simulink model "backstepping_handle_statico_last"  (R2018b)
settings: Solver=VariableStepAuto  StartTime=0.0  StopTime=10  RelTol=1e-3
values from neighbouring files (symbols this model uses):
  cond_init = [0, 150/180*pi, pi/3, -pi/2, -3*pi/4,-150/180*pi]'    [init.m]
  hand_des = p(6,:)'    [init.m]
  Law_param = [kd,kd,kd,kd,kd,kd ... (first row only)    [LAUNCH_Backstepping.m]    (also in LAUNCH_Backstepping_Adaptavive.m = [kp,kp,kp,kp,kp,kp; LAUNCH_PD_TRAJ.m = [300000,300000,300000,300000,300000,300000)
  param = param'    [init.m]
settings Model: Creator=Utente  LastModifiedBy=Utente

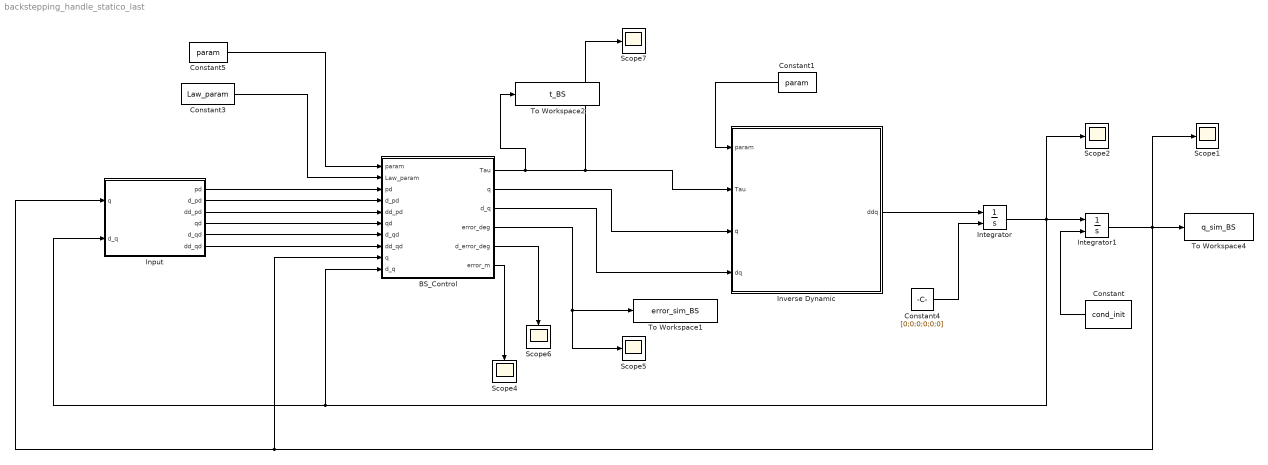
== system backstepping_handle_statico_last ==
  BS_Control : MATLAB Function  TreatAsAtomicUnit=on
  Constant : Constant  Value=cond_init
  Constant1 : Constant  Value=param
  Constant3 : Constant  Value=Law_param
  Constant4 : Constant  Value=[0;0;0;0;0;0]
  Constant5 : Constant  Value=param
  Input : Subsystem
  Integrator : Integrator  InitialConditionSource=external  InitialCondition=[0;0;0;0;0;0]
  Integrator1 : Integrator  InitialConditionSource=external
  Inverse Dynamic : MATLAB Function  TreatAsAtomicUnit=on
  Scope{1..2,4..7} (6 alike) : Scope
  To Workspace1 : ToWorkspace  VariableName=error_sim_BS  SaveFormat=Structure With Time  SampleTime=-1
      settings: Save2DSignal=2-D array (concatenate along first dimension)
  To Workspace2 : ToWorkspace  VariableName=t_BS  SaveFormat=Structure With Time  SampleTime=-1
      settings: Save2DSignal=2-D array (concatenate along first dimension)
  To Workspace4 : ToWorkspace  VariableName=q_sim_BS  SaveFormat=Structure With Time  SampleTime=-1
      settings: Save2DSignal=2-D array (concatenate along first dimension)
  wires:
  Constant5/1 -> BS_Control/1(param)
  Constant3/1 -> BS_Control/2(Law_param)
  BS_Control/2(q) -> Inverse Dynamic/3(q)
  BS_Control/3(d_q) -> Inverse Dynamic/4(dq)
  Constant4/1 -> Integrator/2
  Integrator/1 -> BS_Control/10("d_q "), Input/2(d_q), Integrator1/1, Scope2/1
  Integrator1/1 -> Input/1(q), BS_Control/9("q "), To Workspace4/1, Scope1/1
  Inverse Dynamic/1(ddq) -> Integrator/1
  Constant/1 -> Integrator1/2
  Constant1/1 -> Inverse Dynamic/1(param)
  BS_Control/4(error_deg) -> Scope5/1, To Workspace1/1
  BS_Control/5(d_error_deg) -> Scope6/1
  Input/4(qd) -> BS_Control/6(qd)
  Input/5(d_qd) -> BS_Control/7(d_qd)
  Input/6(dd_qd) -> BS_Control/8(dd_qd)
  Input/3(dd_pd) -> BS_Control/5(dd_pd)
  Input/2(d_pd) -> BS_Control/4(d_pd)
  Input/1(pd) -> BS_Control/3(pd)
  BS_Control/6(error_m) -> Scope4/1
  BS_Control/1(Tau) -> To Workspace2/1, Scope7/1, Inverse Dynamic/2(Tau)

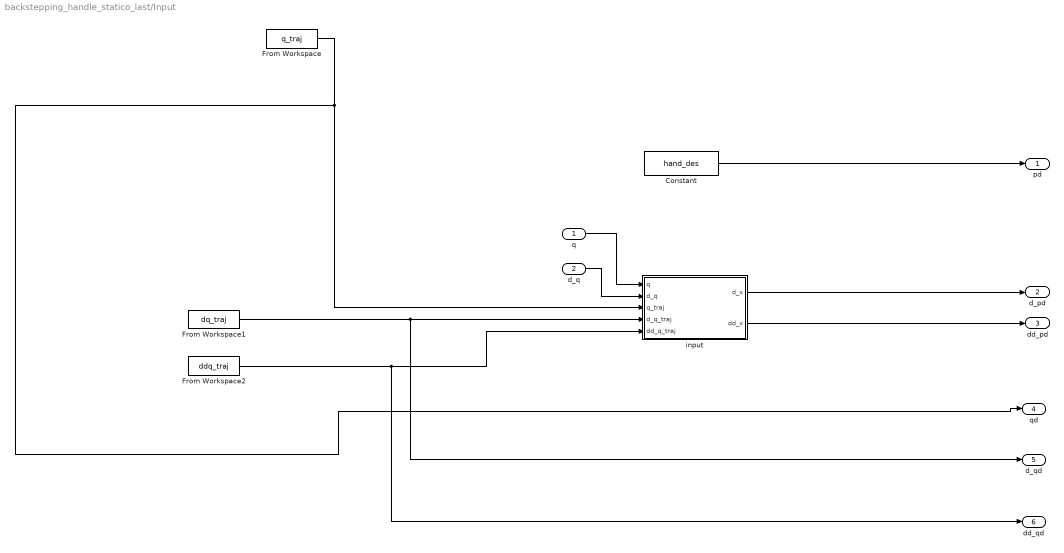
== system backstepping_handle_statico_last/Input ==
  q : Inport
  d_q : Inport  Port=2
  Constant : Constant  Value=hand_des
  From Workspace : FromWorkspace  VariableName=q_traj  SampleTime=0
  From Workspace1 : FromWorkspace  VariableName=dq_traj  SampleTime=0
  From Workspace2 : FromWorkspace  VariableName=ddq_traj  SampleTime=0
  "input " : MATLAB Function  TreatAsAtomicUnit=on
  pd : Outport
  d_pd : Outport  Port=2
  dd_pd : Outport  Port=3
  qd : Outport  Port=4
  d_qd : Outport  Port=5
  dd_qd : Outport  Port=6
  wires:
  From Workspace/1 -> "input "/3(q_traj), qd/1
  From Workspace1/1 -> d_qd/1, "input "/4(d_q_traj)
  From Workspace2/1 -> dd_qd/1, "input "/5(dd_q_traj)
  q/1 -> "input "/1(q)
  d_q/1 -> "input "/2(d_q)
  "input "/1(d_x) -> d_pd/1
  "input "/2(dd_x) -> dd_pd/1
  Constant/1 -> pd/1

== matlab function backstepping_handle_statico_last/BS_Control ==
  data: param input; Tau output; Law_param input; pd input; d_pd input; dd_pd input; qd input; d_qd input; dd_qd input; q input; d_q input; q output; d_q output; error_deg output; d_error_deg output; error_m output
function [Tau, q, d_q, error_deg, d_error_deg, error_m] = BS_Control(param, Law_param, pd, d_pd, dd_pd,qd, d_qd, dd_qd, q, d_q)


    [B,C,G] = Dinamica_new(param,q,d_q);
    
    JHand = J_hand_fun(q);
    pinv_JHand = pinv(JHand);
    
    [p,~,~] = Direct_Kinematics(param,q);
    
    d_Jhand = d_Jhand_fun(q,d_q);
    pinv_d_JHand = pinv(d_Jhand);
    
    Kd = Law_param(1,1)*eye(6);
    L = Law_param(2,1)*eye(6);
    e = qd - q;
    d_e = d_qd - d_q;
    
    d_qr = d_qd + L*e;
    dd_qr = dd_qd + L*d_e;

    s = d_qr - d_q;   
    
    Tau = B*dd_qr + C*d_qr + G + Kd*s + e;

    %SPAZIO TASK
%     Kd = Law_param(1,1)*eye(6);
%     L = Law_param(2,1)*eye(3);
% 
%     e = pd - p(6,:)';
%     d_e = d_pd - JHand*d_q;
%     
%     d_qr = pinv_JHand*(d_pd + L*e);    
%     dd_qr = pinv_JHand*(dd_pd + L*d_e) + pinv_d_JHand*(d_pd + L*e);
% 
%     s = d_qr - d_q;
%     
%     Tau = B*dd_qr + C*d_qr + G + Kd*s + JHand'*e;
    
    error_deg = e*180/pi;
    d_error_deg = d_e*180/pi;
    
    error_m = e;

    
end

== matlab function backstepping_handle_statico_last/Input/input  ==
  data: q input; d_q input; q_traj input; d_x output; d_q_traj input; dd_x output; dd_q_traj input
function [d_x,dd_x] = input_Cond(q, d_q, q_traj, d_q_traj, dd_q_traj)

    JHand = J_hand_fun(q);
    d_JHand = d_Jhand_fun(q,d_q);
    
    d_x = JHand*q_traj;
    dd_x = d_JHand*d_q_traj + JHand*dd_q_traj;
end

== matlab function backstepping_handle_statico_last/Inverse Dynamic ==
  data: param input; Tau input; ddq output; q input; dq input
function ddq = inverseD(param,Tau,q,dq)

    [B,C,G] = Dinamica_new(param,q,dq);
    tot = Tau - C*dq - G;
    
    ddq = B\(tot);
    
end
